simulink model "getGyro"  (R2019a)
settings: Solver=FixedStepAuto  StartTime=0.0  StopTime=inf  RelTol=1e-3  EnableMultiTasking=on
settings Model: SimulationMode=external  Creator=bspoe  LastModifiedBy=florian
settings SolverCC: PositivePriorityOrder=on
settings OptimizationCC: EnhancedBackFolding=on  PassReuseOutputArgsAs=Individual arguments  MaxStackSize=64  OptimizeBlockOrder=speed  DifferentSizesBufferReuse=on  OptimizationCustomize=off
settings DebuggingCC: ParameterTunabilityLossMsg=error
settings HardwareCC: ProdBitPerPointer=32  ProdBitPerSizeT=32  ProdBitPerPtrDiffT=32  ProdLargestAtomicInteger=Long  ProdLargestAtomicFloat=Double  ProdWordSize=32  ProdLongLongMode=on  ProdHWDeviceType=ARM Compatible->ARM Cortex
settings SFSimCC: MATLABDynamicMemAlloc=off
settings RTWCC: SystemTargetFile=ert.tlc  HardwareBoard=Raspberry Pi  TLCOptions="-aInlineSetEventsForThisBaseRateFcn=TLC_FALSE -aSuppressMultiTaskScheduler=TLC_FALSE  -aRateBasedStepFcn=0"  TemplateMakefile=ert_default_tmf  GenerateReport=on  Toolchain=GNU GCC Raspberry Pi  IncludeHyperlinkInReport=on  LaunchReport=on  GenerateTraceInfo=on  GenerateTraceReport=on  GenerateTraceReportSl=on  GenerateTraceReportSf=on  GenerateTraceReportEml=on
settings CodeAppCC: ForceParamTrailComments=on  IgnoreCustomStorageClasses=off  OperatorAnnotations=on  SimulinkDataObjDesc=on  SFDataObjDesc=on  InsertBlockDesc=on
settings ERTTargetCC: SupportContinuousTime=on  SupportVariableSizeSignals=on

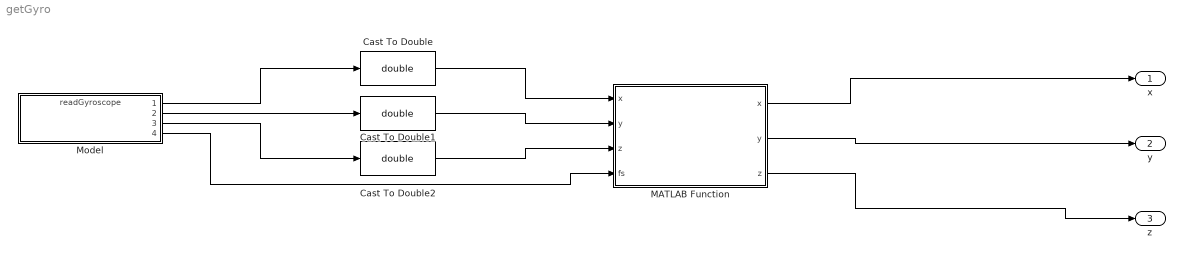
== system getGyro ==
  Cast To Double : DataTypeConversion  OutDataTypeStr=double
  Cast To Double1 : DataTypeConversion  OutDataTypeStr=double
  Cast To Double2 : DataTypeConversion  OutDataTypeStr=double
  MATLAB Function : MATLAB Function  TreatAsAtomicUnit=on
  Model : ModelReference  ModelNameDialog=readGyroscope.slx  SimulationMode=Normal  ModelReferenceVersion=1.9
  x : Outport
  y : Outport  Port=2
  z : Outport  Port=3
  wires:
  Model/1 -> Cast To Double/1
  Model/2 -> Cast To Double1/1
  Model/3 -> Cast To Double2/1
  Cast To Double/1 -> MATLAB Function/1("x ")
  Cast To Double1/1 -> MATLAB Function/2("y ")
  Cast To Double2/1 -> MATLAB Function/3("z ")
  Model/4 -> MATLAB Function/4(fs)
  MATLAB Function/3(z) -> z/1
  MATLAB Function/2(y) -> y/1
  MATLAB Function/1(x) -> x/1

== matlab function getGyro/MATLAB Function ==
  data: x output; x input; y output; y input; z input; fs input; z output
function [x, y, z] = getPhysicalValues(x, y ,z, fs)
    
    sensitivity = 0;
    if fs == 125
        sensitivity = 4.375; 
    elseif fs == 245
         sensitivity = 8.75;
    elseif fs == 500
         sensitivity = 17.5;
    elseif fs == 1000
         sensitivity = 35;
    elseif fs == 2000
         sensitivity = 70;
    end
    
    x = x*sensitivity/1000;
    y = y*sensitivity/1000;
    z = z*sensitivity/1000;
